simulink model "RCAM_model_sim"  (R2025a)
settings: Solver=VariableStepAuto  StartTime=0.0  StopTime=timeFinal  RelTol=1e-3
values from neighbouring files (symbols this model uses):
  amplitud_doblete1 = 7 * pi / 180    (= 0.12217304764)    [inicioWS.m]
  amplitud_doblete2 = 0 * pi / 180    (= 0)    [inicioWS.m]
  amplitud_doblete3 = 0 * pi / 180    (= 0)    [inicioWS.m]
  amplitud_ida_1 = 5 * pi/180    (= 0.0872664625997)    [inicioWS.m]
  amplitud_impulso_1 = 10 * pi/180    (= 0.174532925199)    [inicioWS.m]
  amplitud_impulso_2 = 7 * pi/180    (= 0.12217304764)    [inicioWS.m]
  amplitud_impulso_3 = 0 * pi/180    (= 0)    [inicioWS.m]
  amplitud_impulso_4 = 0 * pi/180    (= 0)    [inicioWS.m]
  amplitud_impulso_5 = 4 * pi/180    (= 0.0698131700798)    [inicioWS.m]
  amplitud_step1 = 0 * pi/180    (= 0)    [inicioWS.m]
  amplitud_step2 = 10.9 * pi/180    (= 0.190240888467)    [inicioWS.m]
  amplitud_step3 = 3 * pi/180    (= 0.0523598775598)    [inicioWS.m]
  amplitud_step4 = 0 * pi/180    (= 0)    [inicioWS.m]
  amplitud_step5 = 0 * pi/180    (= 0)    [inicioWS.m]
  amplitud_vuelta_1 = -amplitud_ida_1 * 2    (= -0.174532925199)    [inicioWS.m]
  duracion_impulso_1 = 6    [inicioWS.m]
  duracion_impulso_2 = 5    [inicioWS.m]
  duracion_impulso_3 = 4    [inicioWS.m]
  duracion_impulso_4 = 4    [inicioWS.m]
  duracion_impulso_5 = 400    [inicioWS.m]
  oei_forzado_value = 0    [inicioWS.m]
  t_doblete_1_p1 = 50    [inicioWS.m]
  t_doblete_1_p2 = t_doblete_1_p1 + 2    (= 52)    [inicioWS.m]
  t_doblete_1_p3 = t_doblete_1_p2 + 1    (= 53)    [inicioWS.m]
  t_doblete_1_p4 = t_doblete_1_p3 + 2    (= 55)    [inicioWS.m]
  t_doblete_2_p1 = 250    [inicioWS.m]
  t_doblete_2_p2 = t_doblete_2_p1 + 3    (= 253)    [inicioWS.m]
  t_doblete_2_p3 = t_doblete_2_p2 + 1    (= 254)    [inicioWS.m]
  t_doblete_2_p4 = t_doblete_2_p3 + 3    (= 257)    [inicioWS.m]
  t_doblete_3_p1 = 200    [inicioWS.m]
  t_doblete_3_p2 = t_doblete_3_p1 + 3    (= 203)    [inicioWS.m]
  t_doblete_3_p3 = t_doblete_3_p2 + 1    (= 204)    [inicioWS.m]
  t_doblete_3_p4 = t_doblete_3_p3 + 3    (= 207)    [inicioWS.m]
  t_impulso_1 = 100    [inicioWS.m]
  t_impulso_2 = 180    [inicioWS.m]
  t_impulso_3 = 300    [inicioWS.m]
  t_impulso_4 = 300    [inicioWS.m]
  t_impulso_5 = 450    [inicioWS.m]
  t_inv_deflex_1_p1 = 100    [inicioWS.m]
  t_inv_deflex_1_p2 = t_inv_deflex_1_p1 + 120    (= 220)    [inicioWS.m]
  t_inv_deflex_1_p3 = t_inv_deflex_1_p2 + 120    (= 340)    [inicioWS.m]
  t_step1 = 250    [inicioWS.m]
  t_step2 = 160    [inicioWS.m]
  t_step3 = 260    [inicioWS.m]
  t_step4 = 8000    [inicioWS.m]
  t_step5 = 420    [inicioWS.m]
  time_oei_forzado_1 = 20000    [inicioWS.m]
  time_oei_forzado_2 = 100    [inicioWS.m]
  u1max = 25*(pi/180)    (= 0.436332312999)    [inicioWS.m]
  u1min = -15*(pi/180)    (= -0.261799387799)    [inicioWS.m]
  u2max = 10*(pi/180)    (= 0.174532925199)    [inicioWS.m]
  u2min = -25*(pi/180)    (= -0.436332312999)    [inicioWS.m]
  u3max = 30*(pi/180)    (= 0.523598775598)    [inicioWS.m]
  u3min = -30*(pi/180)    (= -0.523598775598)    [inicioWS.m]
  u4max = 10*(pi/180)    (= 0.174532925199)    [inicioWS.m]
  u4min = 0    [inicioWS.m]
  u5max = 10*(pi/180)    (= 0.174532925199)    [inicioWS.m]
  u5min = 0*(pi/180)    (= 0)    [inicioWS.m]
  x0 = [84.990252 ... (first row only)    [inicioWS.m]
undefined symbols (not defined in the file or in its folder): amplitud_escalon, amplitud_impulso, duracion_impulso, oei_toggle_2motors, RCAM_model_pdg_rho, t_escalon, t_impulso
libraries: aerolibanimutils x2, aerolibfltsims x2, aerolibatmos2 x1
settings Model: Creator=pablo  LastModifiedBy=pablo

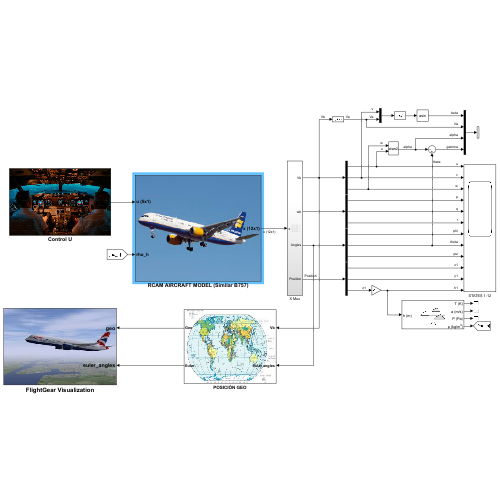
[thumbnail: Simulink's stored preview of the top-level diagram]
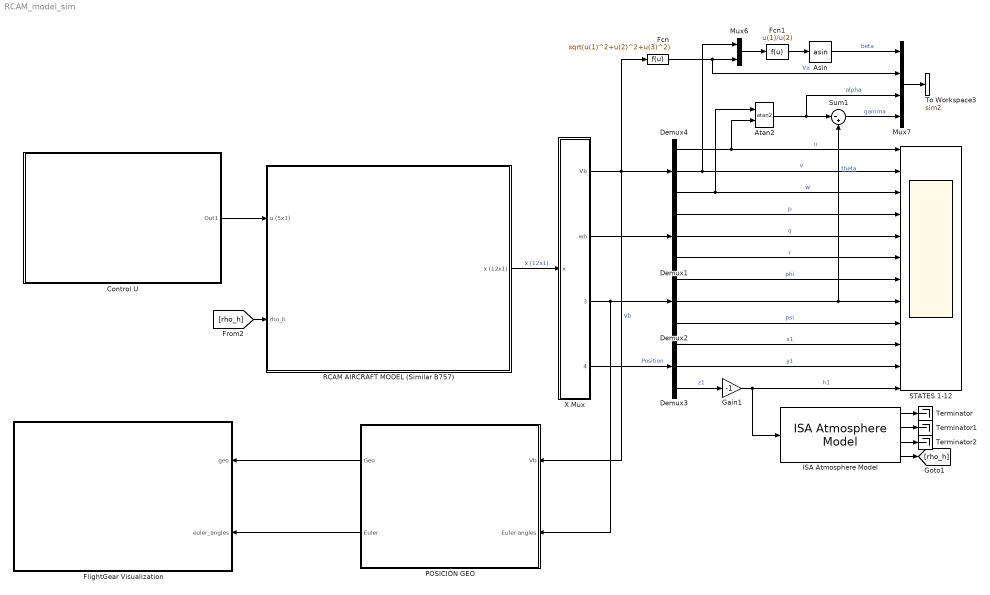
== system RCAM_model_sim ==
  Asin : Trigonometry  Operator=asin
  Atan2 : Trigonometry  Operator=atan2
  Control U : Subsystem
      mask Display: image('descarga3.jpg');
  Demux{1..4} (4 alike) : Demux  Outputs=3
  Fcn : Fcn  Expr=sqrt(u(1)^2+u(2)^2+u(3)^2)
  Fcn1 : Fcn  Expr=u(1)/u(2)
  FlightGear Visualization : Subsystem
      mask Display: image('fg.jpg');
  Gain1 : Gain  Gain=-1
  ISA Atmosphere Model : aerolibatmos2/ISA Atmosphere Model  useExtended=off  action=None  custom=off  viscosityOut=off  g=9.80665  gamma=1.4  R=287.0531  L=0.0065  h_trop=11000  h_strat=20000  rho0=1.225  P0=101325  T0=288.15  h0=0  S=110.4  Tref=273.15  muref=1.716e-5
  Mux6 : Mux  Inputs=2
  Mux7 : Mux
  POSICIÓN GEO : Subsystem
      mask Display: image('descarga.jpg');
  RCAM AIRCRAFT MODEL (Similar B757) : Subsystem
      mask Display: image('zzz.jpg');
  STATES 1-12 : Scope  NumInputPorts=12
      settings: ActiveDisplayYMinimum=80.14131275900877  ActiveDisplayYMaximum=124.43406197108871  DataLoggingVariableName=ScopeData9
  Sum1 : Sum  Inputs=|-+
  Terminator : Terminator
  Terminator1 : Terminator
  Terminator2 : Terminator
  To Workspace3 : ToWorkspace  VariableName=sim2  SaveFormat=Timeseries  SampleTime=-1
  X Mux : Subsystem
  wires:
  RCAM AIRCRAFT MODEL (Similar B757)/1(x (12x1)) -> X Mux/1("x ")  "x (12x1)"
  X Mux/2(wb) -> Demux1/1
  X Mux/4(Position) -> Demux3/1  "Position"
  Control U/1(Out1) -> RCAM AIRCRAFT MODEL (Similar B757)/1(u (5x1))
  X Mux/3(Angles) -> Demux2/1, POSICIÓN GEO/2(Euler angles)
  Atan2/1 -> Sum1/1, Mux7/3  "alpha"
  Sum1/1 -> Mux7/4  "gamma"
  Demux2/2 -> STATES 1-12/8, Sum1/2  "theta"
  Demux2/1 -> STATES 1-12/7  "phi"
  Demux2/3 -> STATES 1-12/9  "psi"
  Demux1/2 -> STATES 1-12/5  "q"
  Demux1/1 -> STATES 1-12/4  "p"
  Demux1/3 -> STATES 1-12/6  "r"
  Demux3/3 -> Gain1/1  "z1"
  Demux3/2 -> STATES 1-12/11  "y1"
  Gain1/1 -> STATES 1-12/12, ISA Atmosphere Model/1  "h1"
  Demux3/1 -> STATES 1-12/10  "x1"
  Fcn/1 -> Mux6/2, Mux7/2  "Va"
  X Mux/1(Vb) -> Fcn/1, Demux4/1, POSICIÓN GEO/1(Vb)  "Vb"
  Mux6/1 -> Fcn1/1
  Fcn1/1 -> Asin/1
  Asin/1 -> Mux7/1  "beta"
  Mux7/1 -> To Workspace3/1
  Demux4/1 -> STATES 1-12/1, Atan2/2  "u"
  Demux4/3 -> STATES 1-12/3, Atan2/1  "w"
  Demux4/2 -> Mux6/1, STATES 1-12/2  "v"
  ISA Atmosphere Model/3 -> Terminator2/1
  ISA Atmosphere Model/2 -> Terminator1/1
  ISA Atmosphere Model/4 -> [rho_h]
  ISA Atmosphere Model/1 -> Terminator/1
  POSICIÓN GEO/1(Geo) -> FlightGear Visualization/1(geo)
  [rho_h] -> RCAM AIRCRAFT MODEL (Similar B757)/2(rho_h)
  POSICIÓN GEO/2(Euler) -> FlightGear Visualization/2(euler_angles)

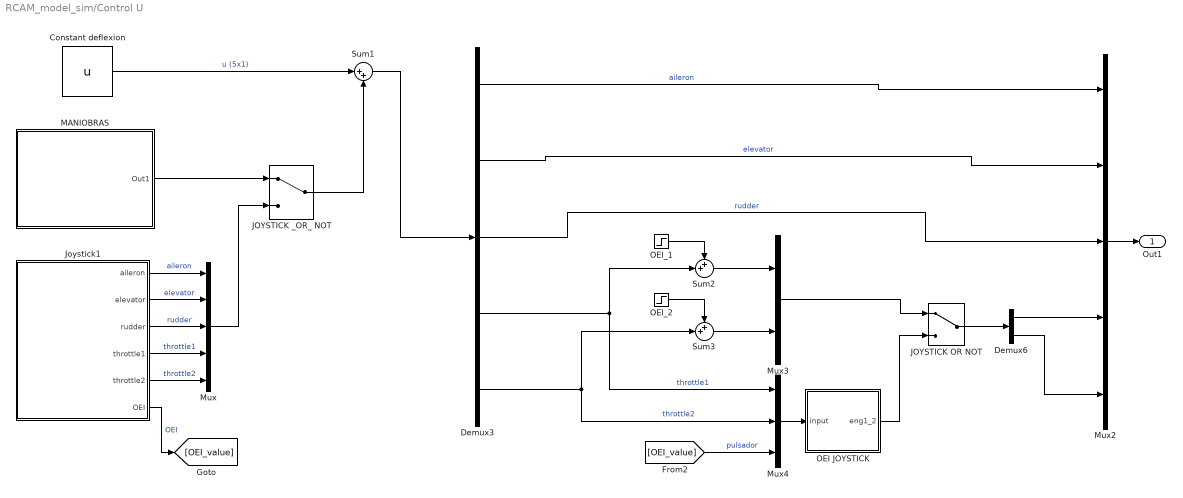
== system RCAM_model_sim/Control U ==
  Constant deflexion : Constant  Value=u  SampleTime=-1
  Demux3 : Demux  Outputs=5
  Demux6 : Demux  Outputs=2
  JOYSTICK OR NOT : ManualSwitch
  JOYSTICK _OR_ NOT : ManualSwitch
  Joystick1 : Subsystem
      mask Display: image('joystick.jpg');
  MANIOBRAS : Subsystem
      mask Display: image('manouverblock.jpg');
  Mux : Mux  Inputs=5
  Mux2 : Mux  Inputs=5
  Mux3 : Mux  Inputs=2
  Mux4 : Mux  Inputs=3
  OEI JOYSTICK : Subsystem
      mask Display: image('OEI.png');
  OEI_1 : Step  Time=time_oei_forzado_1  After=oei_forzado_value  SampleTime=0
  OEI_2 : Step  Time=time_oei_forzado_2  After=oei_forzado_value  SampleTime=0
  Sum1 : Sum  Inputs=|++
  Sum2 : Sum  Inputs=++|
  Sum3 : Sum  Inputs=++|
  Out1 : Outport
  wires:
  Constant deflexion/1 -> Sum1/1  "u (5x1)"
  Joystick1/3(rudder) -> Mux/3  "rudder"
  Joystick1/2(elevator) -> Mux/2  "elevator"
  Joystick1/1(aileron) -> Mux/1  "aileron"
  MANIOBRAS/1(Out1) -> JOYSTICK _OR_ NOT/1
  Mux/1 -> JOYSTICK _OR_ NOT/2
  Joystick1/4(throttle1) -> Mux/4  "throttle1"
  JOYSTICK _OR_ NOT/1 -> Sum1/2
  Joystick1/5(throttle2) -> Mux/5  "throttle2"
  Joystick1/6(OEI) -> [OEI_value]  "OEI"
  Sum1/1 -> Demux3/1
  Demux3/3 -> Mux2/3  "rudder"
  Demux3/1 -> Mux2/1  "aileron"
  Demux3/2 -> Mux2/2  "elevator"
  Demux3/4 -> Mux4/1, Sum2/2  "throttle1"
  Demux3/5 -> Mux4/2, Sum3/2  "throttle2"
  Mux3/1 -> JOYSTICK OR NOT/1
  Mux4/1 -> OEI JOYSTICK/1(input)
  OEI JOYSTICK/1(eng1_2) -> JOYSTICK OR NOT/2
  [OEI_value] -> Mux4/3  "pulsador"
  JOYSTICK OR NOT/1 -> Demux6/1
  Demux6/1 -> Mux2/4
  Demux6/2 -> Mux2/5
  OEI_2/1 -> Sum3/1
  Sum3/1 -> Mux3/2
  OEI_1/1 -> Sum2/1
  Sum2/1 -> Mux3/1
  Mux2/1 -> Out1/1

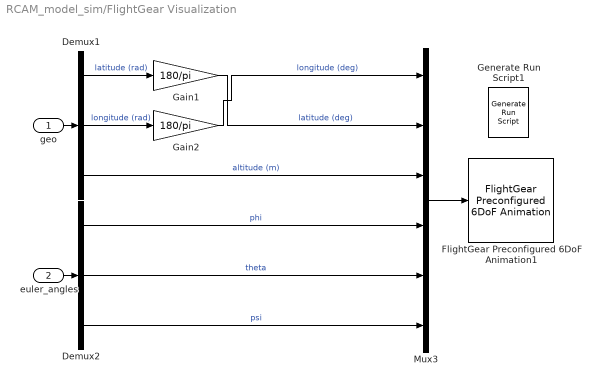
== system RCAM_model_sim/FlightGear Visualization ==
  geo : Inport
  euler_angles : Inport  Port=2
  Demux1 : Demux  Outputs=3
  Demux2 : Demux  Outputs=3
  FlightGear Preconfigured 6DoF Animation1 : aerolibfltsims/FlightGear Preconfigured 6DoF Animation  xFlightGearVersion=v2019.1  DestinationIpAddress=127.0.0.1  DestinationPort=5502  SampleTime=1/30  packetVersion=24
  Gain1 : Gain  Gain=180/pi
  Gain2 : Gain  Gain=180/pi
  Generate Run Script1 : aerolibfltsims/Generate Run Script  Architecture=Default  dataFlow=Send  GeometryModelName=c172p  AirportId=KSFO  RunwayId=10L  InitialAltitude=7224  InitialHeading=113  OffsetDistance=4.72  OffsetAzimuth=0  InstallScenery=off  DisableShaders=on  OriginAddress=127.0.0.1  DestinationPort=5502  OriginPort=5505  LocalAddress=127.0.0.1  OutputFileName=C:\Users\pablo\MATLAB\RCAM_models\BACK_UPPPP\runfg.bat  FlightGearBaseDirectory=C:\Program Files\FlightGear 2024.1
  Mux3 : Mux  Inputs=6
  wires:
  Demux1/3 -> Mux3/3  "altitude (m)"
  Gain1/1 -> Mux3/2  "latitude (deg)"
  Demux1/1 -> Gain1/1  "latitude (rad)"
  Demux1/2 -> Gain2/1  "longitude (rad)"
  Gain2/1 -> Mux3/1  "longitude (deg)"
  Mux3/1 -> FlightGear Preconfigured 6DoF Animation1/1
  geo/1 -> Demux1/1
  euler_angles/1 -> Demux2/1
  Demux2/1 -> Mux3/4  "phi"
  Demux2/2 -> Mux3/5  "theta"
  Demux2/3 -> Mux3/6  "psi"

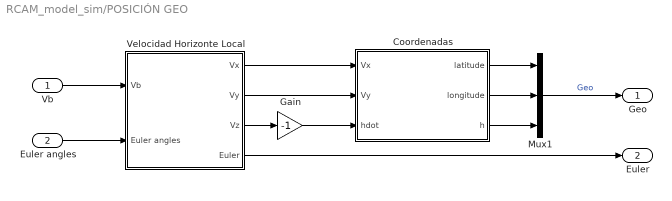
== system RCAM_model_sim/POSICIÓN GEO ==
  Vb : Inport
  Euler angles : Inport  Port=2
  Coordenadas : Subsystem
  Gain : Gain  Gain=-1
  Mux1 : Mux  Inputs=3
  Velocidad Horizonte Local : Subsystem
  Geo : Outport
  Euler : Outport  Port=2
  wires:
  Velocidad Horizonte Local/4(Euler) -> Euler/1
  Coordenadas/2(longitude) -> Mux1/2
  Velocidad Horizonte Local/1(Vx) -> Coordenadas/1(Vx)
  Coordenadas/3(h) -> Mux1/3
  Velocidad Horizonte Local/3(Vz) -> Gain/1
  Velocidad Horizonte Local/2(Vy) -> Coordenadas/2(Vy)
  Coordenadas/1(latitude) -> Mux1/1
  Gain/1 -> Coordenadas/3(hdot)
  Vb/1 -> Velocidad Horizonte Local/1(Vb)
  Euler angles/1 -> Velocidad Horizonte Local/2(Euler angles)
  Mux1/1 -> Geo/1  "Geo"

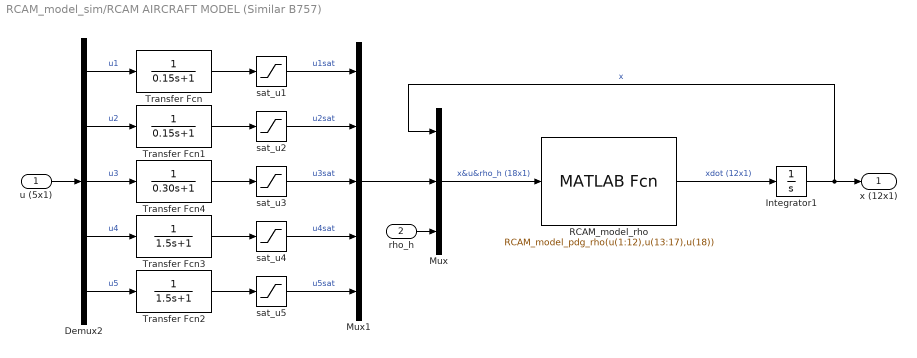
== system RCAM_model_sim/RCAM AIRCRAFT MODEL (Similar B757) ==
  u (5x1) : Inport
  rho_h : Inport  Port=2
  Demux2 : Demux  Outputs=5
  Integrator1 : Integrator  InitialCondition=x0
  Mux : Mux  Inputs=3
  Mux1 : Mux  Inputs=5
  RCAM_model_rho : MATLABFcn  MATLABFcn=RCAM_model_pdg_rho(u(1:12),u(13:17),u(18))
      mask Display: image('descarga (1).jpg');
  Transfer Fcn : TransferFcn  Denominator=[0.15 1]
  Transfer Fcn1 : TransferFcn  Denominator=[0.15 1]
  Transfer Fcn2 : TransferFcn  Denominator=[1.5 1]
  Transfer Fcn3 : TransferFcn  Denominator=[1.5 1]
  Transfer Fcn4 : TransferFcn  Denominator=[0.30 1]
  sat_u1 : Saturate  UpperLimit=u1max  LowerLimit=u1min
  sat_u2 : Saturate  UpperLimit=u2max  LowerLimit=u2min
  sat_u3 : Saturate  UpperLimit=u3max  LowerLimit=u3min
  sat_u4 : Saturate  UpperLimit=u4max  LowerLimit=u4min
  sat_u5 : Saturate  UpperLimit=u5max  LowerLimit=u5min
  x (12x1) : Outport
  wires:
  Integrator1/1 -> x (12x1)/1, Mux/1  "x"
  Mux/1 -> RCAM_model_rho/1  "x&u&rho_h (18x1)"
  RCAM_model_rho/1 -> Integrator1/1  "xdot (12x1)"
  Mux1/1 -> Mux/2
  rho_h/1 -> Mux/3
  Transfer Fcn2/1 -> sat_u5/1
  sat_u1/1 -> Mux1/1  "u1sat"
  Transfer Fcn/1 -> sat_u1/1
  Demux2/2 -> Transfer Fcn1/1  "u2"
  sat_u5/1 -> Mux1/5  "u5sat"
  Demux2/4 -> Transfer Fcn3/1  "u4"
  Demux2/5 -> Transfer Fcn2/1  "u5"
  Demux2/3 -> Transfer Fcn4/1  "u3"
  sat_u4/1 -> Mux1/4  "u4sat"
  Transfer Fcn1/1 -> sat_u2/1
  Demux2/1 -> Transfer Fcn/1  "u1"
  Transfer Fcn3/1 -> sat_u4/1
  u (5x1)/1 -> Demux2/1
  sat_u2/1 -> Mux1/2  "u2sat"
  sat_u3/1 -> Mux1/3  "u3sat"
  Transfer Fcn4/1 -> sat_u3/1

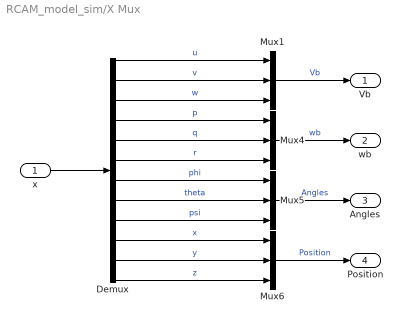
== system RCAM_model_sim/X Mux ==
  "x " : Inport
  Demux : Demux  Outputs=12
  Mux{1,4..6} (4 alike) : Mux  Inputs=3
  Vb : Outport
  wb : Outport  Port=2
  Angles : Outport  Port=3
  Position : Outport  Port=4
  wires:
  Demux/12 -> Mux6/3  "z"
  Mux5/1 -> Angles/1  "Angles"
  Demux/8 -> Mux5/2  "theta"
  Demux/6 -> Mux4/3  "r"
  Demux/11 -> Mux6/2  "y"
  Demux/4 -> Mux4/1  "p"
  Demux/10 -> Mux6/1  "x"
  Demux/5 -> Mux4/2  "q"
  Demux/9 -> Mux5/3  "psi"
  Demux/3 -> Mux1/3  "w"
  Demux/7 -> Mux5/1  "phi"
  Demux/2 -> Mux1/2  "v"
  Demux/1 -> Mux1/1  "u"
  "x "/1 -> Demux/1
  Mux1/1 -> Vb/1  "Vb"
  Mux6/1 -> Position/1  "Position"
  Mux4/1 -> wb/1  "wb"

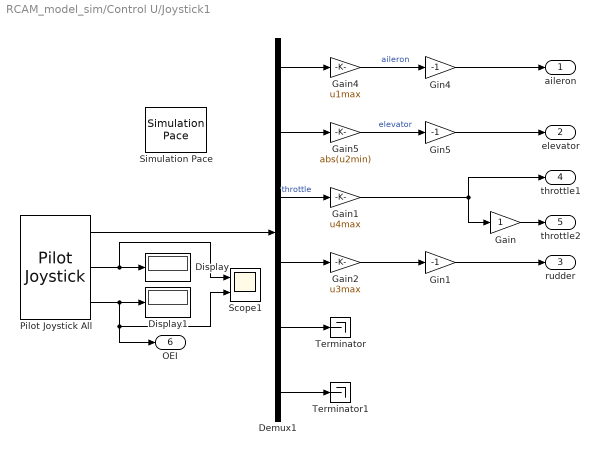
== system RCAM_model_sim/Control U/Joystick1 ==
  Demux1 : Demux  Outputs=6
  Display : Display
      settings: Decimation=5
  Display1 : Display
  Gain : Gain
  Gain1 : Gain  Gain=u4max
  Gain2 : Gain  Gain=u3max
  Gain4 : Gain  Gain=u1max
  Gain5 : Gain  Gain=abs(u2min)
  Gin1 : Gain  Gain=-1
  Gin4 : Gain  Gain=-1
  Gin5 : Gain  Gain=-1
  Pilot Joystick All : aerolibanimutils/Pilot Joystick  JoystickID=Joystick1  OutputConfiguration=AllOutputs  SampleTime=1/30
      settings: LibrarySourceBlock=aerolibanimutils/Pilot Joystick All
  Scope1 : Scope  NumInputPorts=2
      settings: ActiveDisplayYMinimum=55536  ActiveDisplayYMaximum=75536  DataLoggingVariableName=ScopeData15
  Simulation Pace : aerolibanimutils/Simulation Pace  SimulationPace=1  SleepMode=Auto  OutputPaceError=off  SampleTime=1/30
  Terminator : Terminator
  Terminator1 : Terminator
  aileron : Outport
  elevator : Outport  Port=2
  rudder : Outport  Port=3
  throttle1 : Outport  Port=4
  throttle2 : Outport  Port=5
  OEI : Outport  Port=6
  wires:
  Demux1/6 -> Terminator1/1
  Demux1/2 -> Gain5/1
  Demux1/1 -> Gain4/1
  Demux1/3 -> Gain1/1  "throttle"
  Gain5/1 -> Gin5/1  "elevator"
  Gain2/1 -> Gin1/1
  Demux1/5 -> Terminator/1
  Gain4/1 -> Gin4/1  "aileron"
  Demux1/4 -> Gain2/1
  Pilot Joystick All/2 -> Display/1, Scope1/1
  Pilot Joystick All/1 -> Demux1/1
  Pilot Joystick All/3 -> OEI/1, Scope1/2, Display1/1
  Gain/1 -> throttle2/1
  Gain1/1 -> throttle1/1, Gain/1
  Gin4/1 -> aileron/1
  Gin5/1 -> elevator/1
  Gin1/1 -> rudder/1

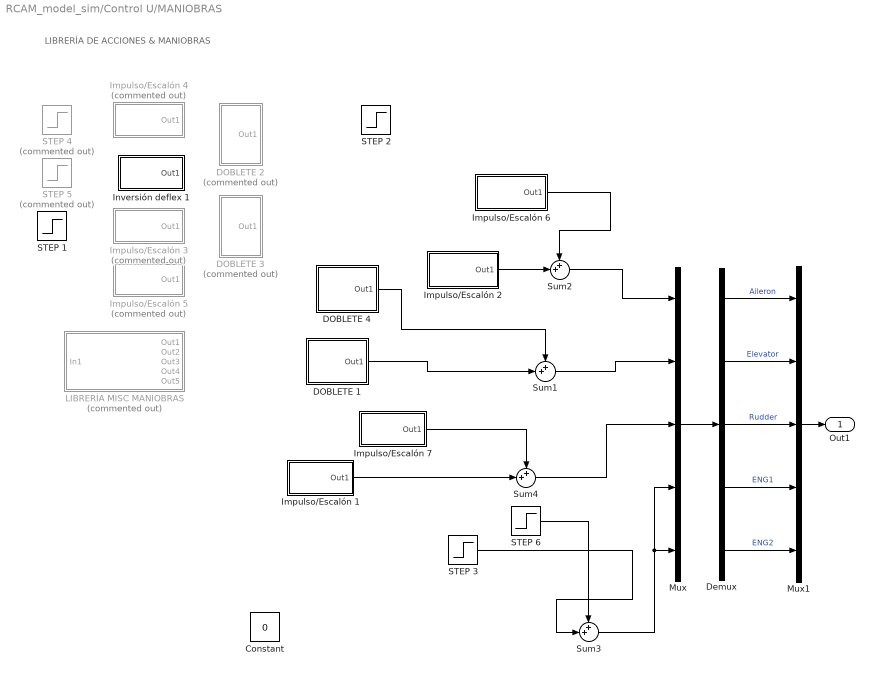
== system RCAM_model_sim/Control U/MANIOBRAS ==
  note: LIBRERÍA DE ACCIONES & MANIOBRAS
  Constant : Constant  Value=0
  DOBLETE 1 : Subsystem
  DOBLETE 2 : Subsystem  Commented=on
  DOBLETE 3 : Subsystem  Commented=on
  DOBLETE 4 : Subsystem
  Demux : Demux  Outputs=5
  Impulso/Escalón 1 : Subsystem
  Impulso/Escalón 2 : Subsystem
  Impulso/Escalón 3 : Subsystem  Commented=on
  Impulso/Escalón 4 : Subsystem  Commented=on
  Impulso/Escalón 5 : Subsystem  Commented=on
  Impulso/Escalón 6 : Subsystem
  Impulso/Escalón 7 : Subsystem
  Inversión deflex 1 : Subsystem
  LIBRERÍA MISC MANIOBRAS : Subsystem  Commented=on
  Mux : Mux  Inputs=5
  Mux1 : Mux  Inputs=5
  STEP 1 : Step  Time=t_step1  After=amplitud_step1  SampleTime=0
  STEP 2 : Step  Time=t_step2  After=amplitud_step2  SampleTime=0
  STEP 3 : Step  Time=t_step3  After=amplitud_step3  SampleTime=0
  STEP 4 : Step  Commented=on  Time=t_step4  After=amplitud_step4  SampleTime=0
  STEP 5 : Step  Commented=on  Time=t_step5  After=amplitud_step5  SampleTime=0
  STEP 6 : Step  Time=360  After=-amplitud_step3  SampleTime=0
  Sum{1..4} (4 alike) : Sum  Inputs=++|
  Out1 : Outport
  wires:
  Impulso/Escalón 1/1(Out1) -> Sum4/2
  DOBLETE 1/1(Out1) -> Sum1/2
  Demux/2 -> Mux1/2  "Elevator"
  Demux/1 -> Mux1/1  "Aileron"
  Demux/3 -> Mux1/3  "Rudder"
  Demux/4 -> Mux1/4  "ENG1"
  Demux/5 -> Mux1/5  "ENG2"
  Mux/1 -> Demux/1
  Mux1/1 -> Out1/1
  STEP 3/1 -> Sum3/2
  Impulso/Escalón 2/1(Out1) -> Sum2/2
  Sum4/1 -> Mux/3
  Sum2/1 -> Mux/1
  Sum1/1 -> Mux/2
  Impulso/Escalón 6/1(Out1) -> Sum2/1
  DOBLETE 4/1(Out1) -> Sum1/1
  Impulso/Escalón 7/1(Out1) -> Sum4/1
  STEP 6/1 -> Sum3/1
  Sum3/1 -> Mux/4, Mux/5

== system RCAM_model_sim/Control U/OEI JOYSTICK ==
  input : Inport
  Interpreted MATLAB Function : MATLABFcn  MATLABFcn=oei_toggle_2motors(u(1),u(2),u(3))
      mask Display: image('OEI.png');
  eng1_2 : Outport
  wires:
  Interpreted MATLAB Function/1 -> eng1_2/1
  input/1 -> Interpreted MATLAB Function/1

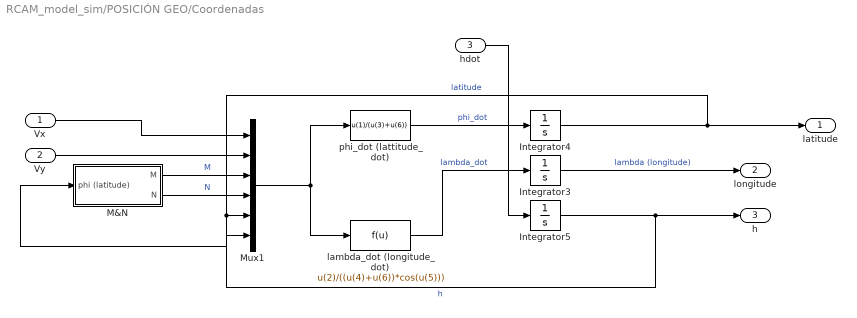
== system RCAM_model_sim/POSICIÓN GEO/Coordenadas ==
  Vx : Inport
  Vy : Inport  Port=2
  hdot : Inport  Port=3
  Integrator3 : Integrator  InitialCondition=1.34
  Integrator4 : Integrator
  Integrator5 : Integrator  InitialCondition=1.3
  M&N : Subsystem
  Mux1 : Mux  Inputs=6
  lambda_dot (longitude_dot) : Fcn  Expr=u(2)/((u(4)+u(6))*cos(u(5)))
  phi_dot (lattitude_dot) : Fcn  Expr=u(1)/(u(3)+u(6))
  latitude : Outport
  longitude : Outport  Port=2
  h : Outport  Port=3
  wires:
  M&N/2(N) -> Mux1/4  "N"
  Vy/1 -> Mux1/2
  phi_dot (lattitude_dot)/1 -> Integrator4/1  "phi_dot"
  Mux1/1 -> lambda_dot (longitude_dot)/1, phi_dot (lattitude_dot)/1
  M&N/1(M) -> Mux1/3  "M"
  Integrator5/1 -> h/1, Mux1/6  "h"
  lambda_dot (longitude_dot)/1 -> Integrator3/1  "lambda_dot"
  Integrator4/1 -> latitude/1, M&N/1(phi (latitude)), Mux1/5  "latitude"
  Vx/1 -> Mux1/1
  hdot/1 -> Integrator5/1
  Integrator3/1 -> longitude/1  "lambda (longitude)"

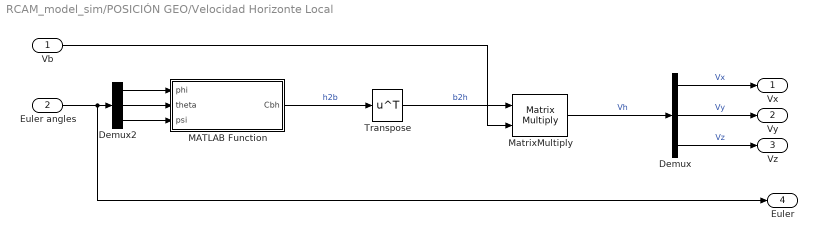
== system RCAM_model_sim/POSICIÓN GEO/Velocidad Horizonte Local ==
  Vb : Inport
  Euler angles : Inport  Port=2
  Demux : Demux  Outputs=3
  Demux2 : Demux  Outputs=3
  MATLAB Function : MATLAB Function  TreatAsAtomicUnit=on
  MatrixMultiply : Product  Multiplication=Matrix(*)
  Transpose : Math  Operator=transpose
  Vx : Outport
  Vy : Outport  Port=2
  Vz : Outport  Port=3
  Euler : Outport  Port=4
  wires:
  Transpose/1 -> MatrixMultiply/1  "b2h"
  MatrixMultiply/1 -> Demux/1  "Vh"
  Demux2/2 -> MATLAB Function/2(theta)
  Demux2/1 -> MATLAB Function/1(phi)
  Demux2/3 -> MATLAB Function/3(psi)
  Vb/1 -> MatrixMultiply/2
  MATLAB Function/1(Cbh) -> Transpose/1  "h2b"
  Demux/1 -> Vx/1  "Vx"
  Demux/2 -> Vy/1  "Vy"
  Demux/3 -> Vz/1  "Vz"
  Euler angles/1 -> Euler/1, Demux2/1

== system RCAM_model_sim/Control U/MANIOBRAS/DOBLETE 1 ==
  Minus4 : Sum  Inputs=++++
  Step33 : Step  Time=t_doblete_1_p1  After=amplitud_doblete1  SampleTime=0
  Step34 : Step  Time=t_doblete_1_p2  After=-amplitud_doblete1  SampleTime=0
  Step36 : Step  Time=t_doblete_1_p3  After=-amplitud_doblete1  SampleTime=0
  Step39 : Step  Time=t_doblete_1_p4  After=amplitud_doblete1  SampleTime=0
  Out1 : Outport
  wires:
  Step36/1 -> Minus4/3
  Step33/1 -> Minus4/1
  Step39/1 -> Minus4/4
  Minus4/1 -> Out1/1
  Step34/1 -> Minus4/2

== system RCAM_model_sim/Control U/MANIOBRAS/DOBLETE 2 ==
  Minus1 : Sum  Inputs=++++
  Step12 : Step  Time=t_doblete_2_p4  After=amplitud_doblete2  SampleTime=0
  Step4 : Step  Time=t_doblete_2_p1  After=amplitud_doblete2  SampleTime=0
  Step7 : Step  Time=t_doblete_2_p2  After=-amplitud_doblete2  SampleTime=0
  Step8 : Step  Time=t_doblete_2_p3  After=-amplitud_doblete2  SampleTime=0
  Out1 : Outport
  wires:
  Step4/1 -> Minus1/1
  Step12/1 -> Minus1/4
  Step7/1 -> Minus1/2
  Step8/1 -> Minus1/3
  Minus1/1 -> Out1/1

== system RCAM_model_sim/Control U/MANIOBRAS/DOBLETE 3 ==
  Minus1 : Sum  Inputs=++++
  Step12 : Step  Time=t_doblete_3_p4  After=amplitud_doblete3  SampleTime=0
  Step4 : Step  Time=t_doblete_3_p1  After=amplitud_doblete3  SampleTime=0
  Step7 : Step  Time=t_doblete_3_p2  After=-amplitud_doblete3  SampleTime=0
  Step8 : Step  Time=t_doblete_3_p3  After=-amplitud_doblete3  SampleTime=0
  Out1 : Outport
  wires:
  Step4/1 -> Minus1/1
  Step12/1 -> Minus1/4
  Step7/1 -> Minus1/2
  Step8/1 -> Minus1/3
  Minus1/1 -> Out1/1

== system RCAM_model_sim/Control U/MANIOBRAS/DOBLETE 4 ==
  Minus4 : Sum  Inputs=++++
  Step33 : Step  Time=450  After=amplitud_doblete1  SampleTime=0
  Step34 : Step  Time=450+2  After=-amplitud_doblete1  SampleTime=0
  Step36 : Step  Time=450+3  After=-amplitud_doblete1  SampleTime=0
  Step39 : Step  Time=450+2  After=amplitud_doblete1  SampleTime=0
  Out1 : Outport
  wires:
  Step36/1 -> Minus4/3
  Step33/1 -> Minus4/1
  Step39/1 -> Minus4/4
  Minus4/1 -> Out1/1
  Step34/1 -> Minus4/2

== system RCAM_model_sim/Control U/MANIOBRAS/Impulso//Escalón 1 ==
  Step13 : Step  Time=t_impulso_1  After=amplitud_impulso_1  SampleTime=0
  Step38 : Step  Time=t_impulso_1+duracion_impulso_1  After=-amplitud_impulso_1  SampleTime=0
  Sum1 : Sum  Inputs=++|
  Out1 : Outport
  wires:
  Sum1/1 -> Out1/1
  Step38/1 -> Sum1/2
  Step13/1 -> Sum1/1

== system RCAM_model_sim/Control U/MANIOBRAS/Impulso//Escalón 2 ==
  Step14 : Step  Time=550  After=amplitud_impulso_2  SampleTime=0
  Step15 : Step  Time=555  After=-amplitud_impulso_2  SampleTime=0
  Sum5 : Sum  Inputs=++|
  Out1 : Outport
  wires:
  Step14/1 -> Sum5/1
  Step15/1 -> Sum5/2
  Sum5/1 -> Out1/1

== system RCAM_model_sim/Control U/MANIOBRAS/Impulso//Escalón 3 ==
  Step4 : Step  Time=t_impulso_3  After=amplitud_impulso_3  SampleTime=0
  Step7 : Step  Time=t_impulso_3+duracion_impulso_3  After=-amplitud_impulso_3  SampleTime=0
  Sum3 : Sum  Inputs=++|
  Out1 : Outport
  wires:
  Sum3/1 -> Out1/1
  Step4/1 -> Sum3/1
  Step7/1 -> Sum3/2

== system RCAM_model_sim/Control U/MANIOBRAS/Impulso//Escalón 4 ==
  Step12 : Step  Time=t_impulso_4+duracion_impulso_4  After=-amplitud_impulso_4  SampleTime=0
  Step8 : Step  Time=t_impulso_4  After=amplitud_impulso_4  SampleTime=0
  Sum4 : Sum  Inputs=++|
  Out1 : Outport
  wires:
  Step12/1 -> Sum4/2
  Step8/1 -> Sum4/1
  Sum4/1 -> Out1/1

== system RCAM_model_sim/Control U/MANIOBRAS/Impulso//Escalón 5 ==
  Step12 : Step  Time=t_impulso_5+duracion_impulso_5  After=-amplitud_impulso_5  SampleTime=0
  Step8 : Step  Time=t_impulso_5  After=amplitud_impulso_5  SampleTime=0
  Sum4 : Sum  Inputs=++|
  Out1 : Outport
  wires:
  Step12/1 -> Sum4/2
  Step8/1 -> Sum4/1
  Sum4/1 -> Out1/1

== system RCAM_model_sim/Control U/MANIOBRAS/Impulso//Escalón 6 ==
  Step14 : Step  Time=t_impulso_2  After=amplitud_impulso_2  SampleTime=0
  Step15 : Step  Time=t_impulso_2+duracion_impulso_2  After=-amplitud_impulso_2  SampleTime=0
  Sum5 : Sum  Inputs=++|
  Out1 : Outport
  wires:
  Step14/1 -> Sum5/1
  Step15/1 -> Sum5/2
  Sum5/1 -> Out1/1

== system RCAM_model_sim/Control U/MANIOBRAS/Impulso//Escalón 7 ==
  Step13 : Step  Time=630  After=amplitud_impulso_1  SampleTime=0
  Step38 : Step  Time=635  After=-amplitud_impulso_1  SampleTime=0
  Sum1 : Sum  Inputs=++|
  Out1 : Outport
  wires:
  Sum1/1 -> Out1/1
  Step38/1 -> Sum1/2
  Step13/1 -> Sum1/1

== system RCAM_model_sim/Control U/MANIOBRAS/Inversión deflex 1 ==
  STEP 6 : Step  Time=t_inv_deflex_1_p3  After=amplitud_ida_1  SampleTime=0
  Step13 : Step  Time=t_inv_deflex_1_p1  After=amplitud_ida_1  SampleTime=0
  Step38 : Step  Time=t_inv_deflex_1_p2  After=amplitud_vuelta_1  SampleTime=0
  Sum1 : Sum  Inputs=+++
  Out1 : Outport
  wires:
  Sum1/1 -> Out1/1
  Step38/1 -> Sum1/2
  Step13/1 -> Sum1/1
  STEP 6/1 -> Sum1/3

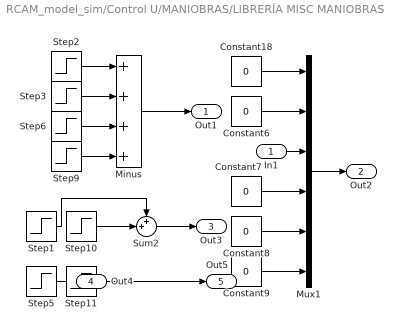
== system RCAM_model_sim/Control U/MANIOBRAS/LIBRERÍA MISC MANIOBRAS ==
  In1 : Inport
  Constant{6..9,18} (5 alike) : Constant  Value=0
  Minus : Sum  Inputs=++++
  Mux1 : Mux  Inputs=6
  Step1 : Step  Time=t_impulso  After=amplitud_impulso  SampleTime=0
  Step10 : Step  Time=t_impulso+duracion_impulso  After=-amplitud_impulso  SampleTime=0
  Step11 : Step  Time=t_escalon  After=amplitud_escalon  SampleTime=0
  Step2 : Step  Time=150  After=5*pi/180  SampleTime=0
  Step3 : Step  Time=300+2  After=-5*pi/180  SampleTime=0
  Step5 : Step  Time=40  After=6*pi/180  SampleTime=0
  Step6 : Step  Time=300+4  After=-5*pi/180  SampleTime=0
  Step9 : Step  Time=300+6  After=5*pi/180  SampleTime=0
  Sum2 : Sum  Inputs=++|
  Out1 : Outport
  Out2 : Outport  Port=2
  Out3 : Outport  Port=3
  Out4 : Outport  Port=4
  Out5 : Outport  Port=5
  wires:
  Step9/1 -> Minus/4
  Step2/1 -> Minus/1
  Constant7/1 -> Mux1/4
  Constant9/1 -> Mux1/6
  Step6/1 -> Minus/3
  Step3/1 -> Minus/2
  Constant6/1 -> Mux1/2
  Constant18/1 -> Mux1/1
  Step11/1 -> Out5/1
  Constant8/1 -> Mux1/5
  Step1/1 -> Sum2/1
  Step10/1 -> Sum2/2
  Mux1/1 -> Out2/1
  In1/1 -> Mux1/3
  Step5/1 -> Out4/1
  Minus/1 -> Out1/1
  Sum2/1 -> Out3/1

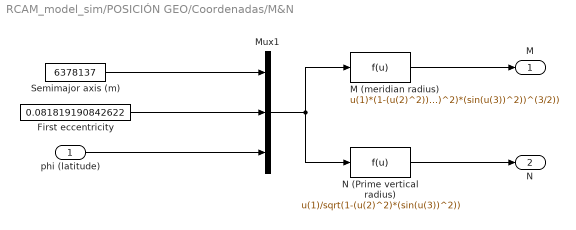
== system RCAM_model_sim/POSICIÓN GEO/Coordenadas/M&N ==
  phi (latitude) : Inport
  First eccentricity : Constant  Value=0.081819190842622
  M (meridian radius) : Fcn  Expr=u(1)*(1-(u(2)^2))/((1-(u(2)^2)*(sin(u(3))^2))^(3/2))
  Mux1 : Mux  Inputs=3
  N (Prime vertical radius) : Fcn  Expr=u(1)/sqrt(1-(u(2)^2)*(sin(u(3))^2))
  Semimajor axis (m) : Constant  Value=6378137
  M : Outport
  N : Outport  Port=2
  wires:
  First eccentricity/1 -> Mux1/2
  M (meridian radius)/1 -> M/1
  Mux1/1 -> N (Prime vertical radius)/1, M (meridian radius)/1
  phi (latitude)/1 -> Mux1/3
  N (Prime vertical radius)/1 -> N/1
  Semimajor axis (m)/1 -> Mux1/1

== matlab function RCAM_model_sim/POSICIÓN GEO/Velocidad Horizonte Local/MATLAB Function ==
  data: phi input; Cbh output; theta input; psi input
function Cbh  = Matriz_h2b(phi, theta, psi)
% DCM_B_TO_V  Direction Cosine Matrix de cuerpo (b) a v (navegación)
% Entradas:  phi (roll), theta (pitch), psi (yaw)   [rad]
% Salidas:   Cbv  (3x3) tal que  v = Cbv * b
%            Cvb  = Cbv'  (de v a b)

cphi = cos(phi);  sphi = sin(phi);
cthe = cos(theta); sthe = sin(theta);
cpsi = cos(psi);  spsi = sin(psi);

Cbh = [ ...
   cthe*cpsi,                      cthe*spsi,                    -sthe; 
  -sphi*sthe*cpsi - cphi*spsi,    -sphi*sthe*spsi + cphi*cpsi,   sphi*cthe;
  -sphi*spsi + cphi*sthe*cpsi,     sphi*cpsi + cphi*sthe*spsi,   cphi*cthe]; 

end
